simulink model "add_dma"  (R2020a)
settings: Solver=FixedStepDiscrete  StartTime=0.0  StopTime=10.0  RelTol=1e-3
libraries: hdlsllib x2
settings Model: DataTypeOverride=Off  Creator=sunip  LastModifiedBy=sunip
settings OptimizationCC: BlockReduction=off  ConditionallyExecuteInputs=off  DefaultParameterBehavior=Inlined  SimCompilerOptimization=on
settings DebuggingCC: AlgebraicLoopMsg=error  SingleTaskRateTransMsg=error
settings HardwareCC: ProdBitPerPointer=32  ProdBitPerSizeT=32  ProdBitPerPtrDiffT=32  ProdLargestAtomicFloat=None  ProdIntDivRoundTo=Undefined  ProdEndianess=Unspecified  ProdWordSize=32  ProdHWDeviceType=ASIC/FPGA->ASIC/FPGA  TargetBitPerLong=64  TargetBitPerPointer=64  TargetBitPerSizeT=64  TargetBitPerPtrDiffT=64  TargetLongLongMode=on  TargetIntDivRoundTo=Zero  TargetEndianess=LittleEndian  TargetWordSize=64  TargetHWDeviceType=Custom Processor->MATLAB Host Computer  ProdEqTarget=off

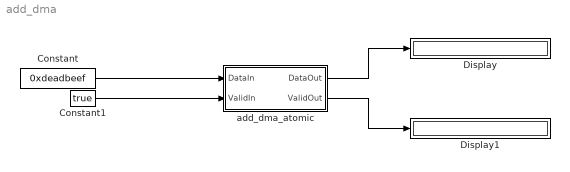
== system add_dma ==
  Constant : Constant  Value=0xdeadbeef  OutDataTypeStr=uint32  SampleTime=-1
  Constant1 : Constant  Value=true
  Display : Display
      settings: Format=hex (Stored Integer)
  Display1 : Display
      settings: Format=binary (Stored Integer)
  add_dma_atomic : Subsystem  TreatAsAtomicUnit=on
  wires:
  Constant/1 -> add_dma_atomic/1(DataIn)
  Constant1/1 -> add_dma_atomic/2(ValidIn)
  add_dma_atomic/1(DataOut) -> Display/1
  add_dma_atomic/2(ValidOut) -> Display1/1

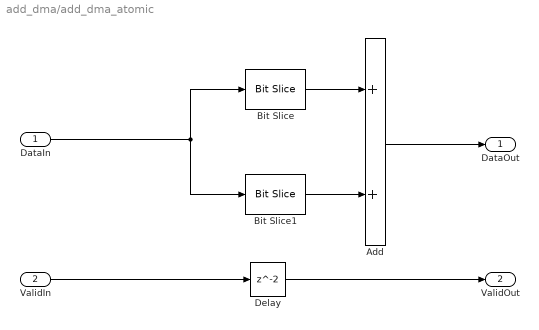
== system add_dma/add_dma_atomic ==
  DataIn : Inport  OutDataTypeStr=uint32  SampleTime=0.001
  ValidIn : Inport  Port=2  OutDataTypeStr=boolean  SampleTime=0.001
  Add : Sum  AccumDataTypeStr=uint32  OutDataTypeStr=uint32
  Bit Slice : hdlsllib/Logic and Bit Operations/Bit Slice  lidx=31  ridx=16
      settings: SourceProductBaseCode=SL
  Bit Slice1 : hdlsllib/Logic and Bit Operations/Bit Slice  lidx=15  ridx=0
      settings: SourceProductBaseCode=SL
  Delay : Delay
  DataOut : Outport  OutDataTypeStr=uint32
  ValidOut : Outport  Port=2  OutDataTypeStr=boolean
  wires:
  Bit Slice1/1 -> Add/2
  DataIn/1 -> Bit Slice/1, Bit Slice1/1
  ValidIn/1 -> Delay/1
  Add/1 -> DataOut/1
  Bit Slice/1 -> Add/1
  Delay/1 -> ValidOut/1
